simulink model "pwm_test"  (R2021b)
settings: Solver=VariableStepAuto  StartTime=0.0  StopTime=0.01  RelTol=1e-3
libraries: spsOnDelayLib x14, simulink x13
settings Model: SimulationMode=accelerator  PacingRate=1000  Creator=phddk  LastModifiedBy=phddk

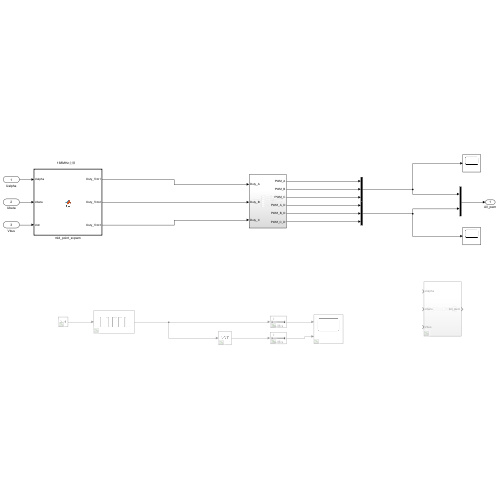
[thumbnail: Simulink's stored preview of the top-level diagram]
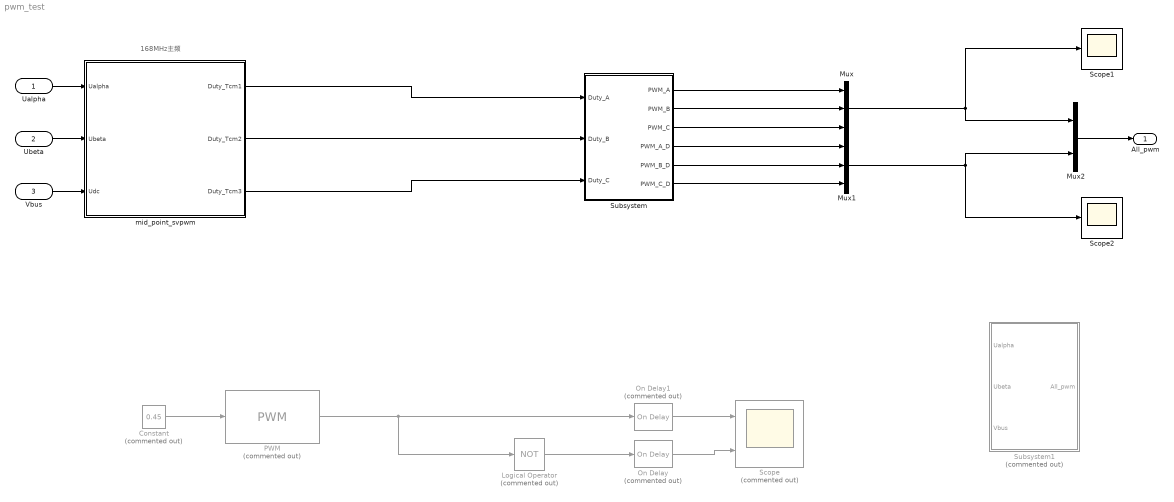
== system pwm_test ==
  note: 168MHz主频
  Ualpha : Inport
  Ubeta : Inport  Port=2
  Vbus : Inport  Port=3
  Constant : Constant  Commented=on  Value=0.45
  Logical Operator : Logic  Commented=on  Operator=NOT  AllPortsSameDT=off  OutDataTypeStr=boolean
  Mux : Mux  Inputs=3
  Mux1 : Mux  Inputs=3
  Mux2 : Mux  Inputs=2
  On Delay : spsOnDelayLib/On Delay  Commented=on  DelayType=On delay  delay=5e-6  ic=0  Ts=0
      settings: SourceProductBaseCode=PS
  On Delay1 : spsOnDelayLib/On Delay  Commented=on  DelayType=On delay  delay=5e-6  ic=0  Ts=0
      settings: SourceProductBaseCode=PS
  PWM : simulink/Discontinuities/PWM  Commented=on  DisableCoverage=on  Period=5e-4  DisallowZeroDutyCycle=off  RunAtFixedTimeIntervals=on  SampleTime=5e-5
  Scope : Scope  Commented=on  NumInputPorts=2
  Scope1 : Scope
  Scope2 : Scope
  Subsystem : Subsystem
  Subsystem1 : Subsystem  Commented=on
  mid_point_svpwm : MATLAB Function  TreatAsAtomicUnit=on
  All_pwm : Outport
  wires:
  On Delay1/1 -> Scope/1
  On Delay/1 -> Scope/2
  Logical Operator/1 -> On Delay/1
  Constant/1 -> PWM/1
  PWM/1 -> Logical Operator/1, On Delay1/1
  mid_point_svpwm/1(Duty_Tcm1) -> Subsystem/1(Duty_A)
  mid_point_svpwm/2(Duty_Tcm2) -> Subsystem/2(Duty_B)
  mid_point_svpwm/3(Duty_Tcm3) -> Subsystem/3(Duty_C)
  Mux/1 -> Mux2/1, Scope1/1
  Subsystem/1(PWM_A) -> Mux/1
  Subsystem/2(PWM_B) -> Mux/2
  Subsystem/3(PWM_C) -> Mux/3
  Subsystem/4(PWM_A_D) -> Mux1/1
  Subsystem/5(PWM_B_D) -> Mux1/2
  Subsystem/6(PWM_C_D) -> Mux1/3
  Mux1/1 -> Scope2/1, Mux2/2
  Mux2/1 -> All_pwm/1
  Ualpha/1 -> mid_point_svpwm/1(Ualpha)
  Ubeta/1 -> mid_point_svpwm/2(Ubeta)
  Vbus/1 -> mid_point_svpwm/3(Udc)

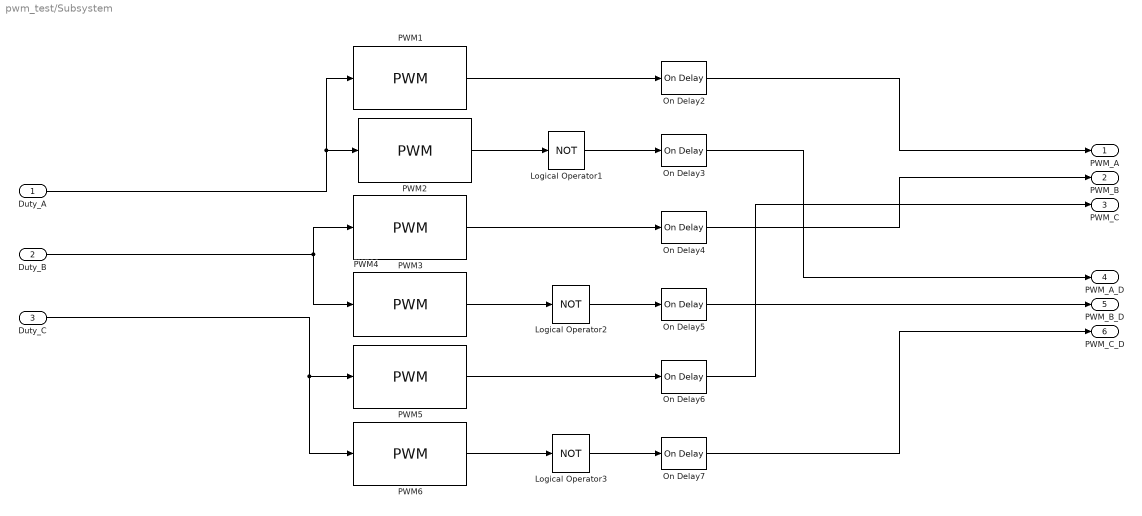
== system pwm_test/Subsystem ==
  Duty_A : Inport
  Duty_B : Inport  Port=2
  Duty_C : Inport  Port=3
  Logical Operator1 : Logic  Operator=NOT  AllPortsSameDT=off  OutDataTypeStr=boolean
  Logical Operator2 : Logic  Operator=NOT  AllPortsSameDT=off  OutDataTypeStr=boolean
  Logical Operator3 : Logic  Operator=NOT  AllPortsSameDT=off  OutDataTypeStr=boolean
  On Delay{2..7} (6 alike) : spsOnDelayLib/On Delay  DelayType=On delay  delay=5e-6  ic=0  Ts=0
      settings: SourceProductBaseCode=PS
  PWM{1..6} (6 alike) : simulink/Discontinuities/PWM  DisableCoverage=on  Period=5e-4  DisallowZeroDutyCycle=off  RunAtFixedTimeIntervals=on  SampleTime=5e-5
  PWM_A : Outport
  PWM_B : Outport  Port=2
  PWM_C : Outport  Port=3
  PWM_A_D : Outport  Port=4
  PWM_B_D : Outport  Port=5
  PWM_C_D : Outport  Port=6
  wires:
  Logical Operator1/1 -> On Delay3/1
  PWM4/1 -> Logical Operator2/1
  Logical Operator2/1 -> On Delay5/1
  Logical Operator3/1 -> On Delay7/1
  PWM6/1 -> Logical Operator3/1
  PWM2/1 -> Logical Operator1/1
  PWM3/1 -> On Delay4/1
  PWM1/1 -> On Delay2/1
  On Delay2/1 -> PWM_A/1
  Duty_A/1 -> PWM1/1, PWM2/1
  Duty_C/1 -> PWM6/1, PWM5/1
  Duty_B/1 -> PWM3/1, PWM4/1
  PWM5/1 -> On Delay6/1
  On Delay4/1 -> PWM_B/1
  On Delay6/1 -> PWM_C/1
  On Delay5/1 -> PWM_B_D/1
  On Delay7/1 -> PWM_C_D/1
  On Delay3/1 -> PWM_A_D/1

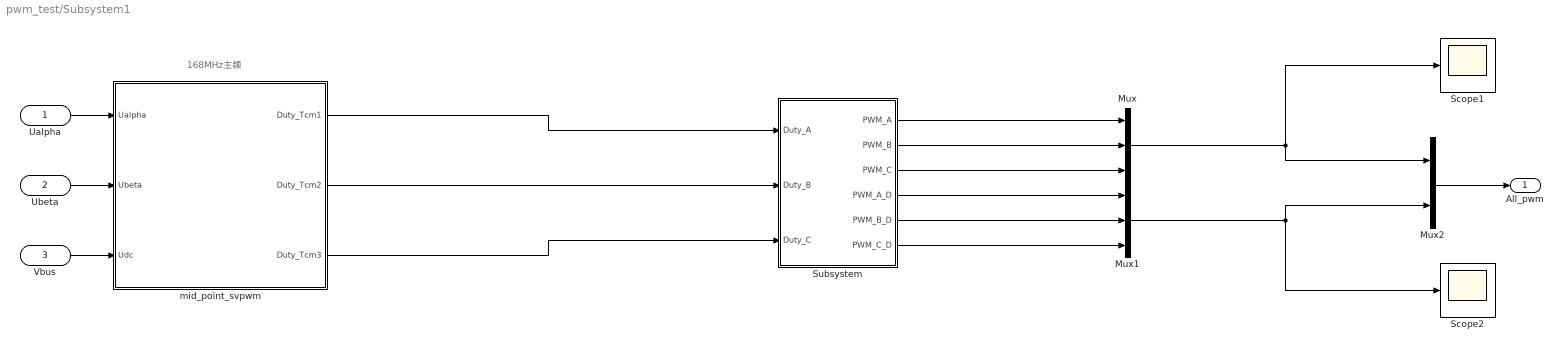
== system pwm_test/Subsystem1 ==
  note: 168MHz主频
  Ualpha : Inport
  Ubeta : Inport  Port=2
  Vbus : Inport  Port=3
  Mux : Mux  Inputs=3
  Mux1 : Mux  Inputs=3
  Mux2 : Mux  Inputs=2
  Scope1 : Scope
  Scope2 : Scope
  Subsystem : Subsystem
  mid_point_svpwm : MATLAB Function  TreatAsAtomicUnit=on
  All_pwm : Outport
  wires:
  Ubeta/1 -> mid_point_svpwm/2(Ubeta)
  Mux2/1 -> All_pwm/1
  Mux/1 -> Mux2/1, Scope1/1
  Subsystem/3(PWM_C) -> Mux/3
  Mux1/1 -> Scope2/1, Mux2/2
  mid_point_svpwm/1(Duty_Tcm1) -> Subsystem/1(Duty_A)
  mid_point_svpwm/2(Duty_Tcm2) -> Subsystem/2(Duty_B)
  mid_point_svpwm/3(Duty_Tcm3) -> Subsystem/3(Duty_C)
  Subsystem/5(PWM_B_D) -> Mux1/2
  Ualpha/1 -> mid_point_svpwm/1(Ualpha)
  Vbus/1 -> mid_point_svpwm/3(Udc)
  Subsystem/4(PWM_A_D) -> Mux1/1
  Subsystem/1(PWM_A) -> Mux/1
  Subsystem/6(PWM_C_D) -> Mux1/3
  Subsystem/2(PWM_B) -> Mux/2

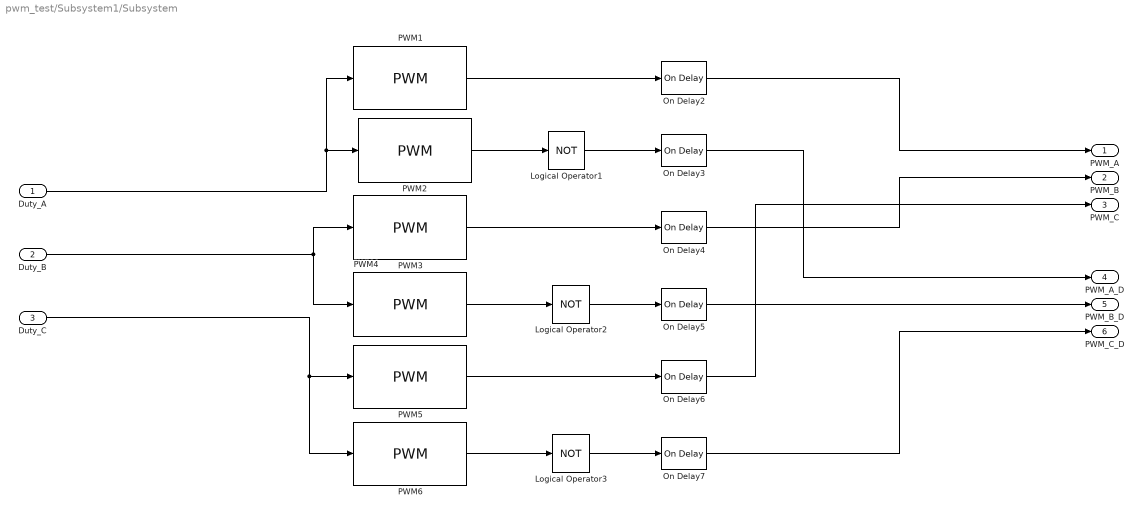
== system pwm_test/Subsystem1/Subsystem ==
  Duty_A : Inport
  Duty_B : Inport  Port=2
  Duty_C : Inport  Port=3
  Logical Operator1 : Logic  Operator=NOT  AllPortsSameDT=off  OutDataTypeStr=boolean
  Logical Operator2 : Logic  Operator=NOT  AllPortsSameDT=off  OutDataTypeStr=boolean
  Logical Operator3 : Logic  Operator=NOT  AllPortsSameDT=off  OutDataTypeStr=boolean
  On Delay{2..7} (6 alike) : spsOnDelayLib/On Delay  DelayType=On delay  delay=5e-6  ic=0  Ts=0
      settings: SourceProductBaseCode=PS
  PWM{1..6} (6 alike) : simulink/Discontinuities/PWM  DisableCoverage=on  Period=5e-4  DisallowZeroDutyCycle=off  RunAtFixedTimeIntervals=on  SampleTime=5e-5
  PWM_A : Outport
  PWM_B : Outport  Port=2
  PWM_C : Outport  Port=3
  PWM_A_D : Outport  Port=4
  PWM_B_D : Outport  Port=5
  PWM_C_D : Outport  Port=6
  wires:
  Logical Operator1/1 -> On Delay3/1
  PWM4/1 -> Logical Operator2/1
  Logical Operator2/1 -> On Delay5/1
  Logical Operator3/1 -> On Delay7/1
  PWM6/1 -> Logical Operator3/1
  PWM2/1 -> Logical Operator1/1
  PWM3/1 -> On Delay4/1
  PWM1/1 -> On Delay2/1
  On Delay2/1 -> PWM_A/1
  Duty_A/1 -> PWM1/1, PWM2/1
  Duty_C/1 -> PWM6/1, PWM5/1
  Duty_B/1 -> PWM3/1, PWM4/1
  PWM5/1 -> On Delay6/1
  On Delay4/1 -> PWM_B/1
  On Delay6/1 -> PWM_C/1
  On Delay5/1 -> PWM_B_D/1
  On Delay7/1 -> PWM_C_D/1
  On Delay3/1 -> PWM_A_D/1

== matlab function pwm_test/mid_point_svpwm ==
  data: Ualpha input; Duty_Tcm1 output; Ubeta input; Udc input; Duty_Tcm2 output; Duty_Tcm3 output
function [Duty_Tcm1,Duty_Tcm2,Duty_Tcm3] = fcn(Ualpha,Ubeta,Udc)
Tcm1 = 0;
Tcm2 = 0;
Tcm3 = 0;

Duty_Tcm1 = 0;
Duty_Tcm2 = 0;
Duty_Tcm3 = 0;


Vmax_pu=0;
Vmin_pu=0;
Vcom_pu=0;

Valpha_pu = Ualpha/Udc;
Vbeta_pu = Ubeta/Udc;
	
Va_tmp = 0.5 * Valpha_pu;
Vb_tmp = 0.8660254038 * Vbeta_pu;

Va_pu = Valpha_pu;
Vb_pu = -Va_tmp + Vb_tmp;						
Vc_pu = -Va_tmp - Vb_tmp;						

if(Va_pu > Vb_pu)
    Vmax_pu = Va_pu;
    Vmin_pu = Vb_pu;
end

if(Va_pu <= Vb_pu)
    Vmax_pu = Vb_pu;
    Vmin_pu = Va_pu;
end

if(Vc_pu > Vmax_pu)
    Vmax_pu = Vc_pu;
end
if(Vc_pu < Vmin_pu)
    Vmin_pu = Vc_pu;
end

Vcom_pu = 0.5 * (Vmax_pu + Vmin_pu);			
	
Tcm1 = (Va_pu - Vcom_pu);
Tcm2 = (Vb_pu - Vcom_pu);
Tcm3 = (Vc_pu - Vcom_pu);

if(Tcm1 > 0.5)
    Tcm1 = 0.5;
end
if(Tcm1 < -0.5)
    Tcm1 = -0.5;
end


if(Tcm2 > 0.5)
    Tcm2 = 0.5;
end
if(Tcm2 < -0.5)
    Tcm2 = -0.5;
end


if(Tcm3 > 0.5)
    Tcm3 = 0.5;
end
if(Tcm3 < -0.5)
    Tcm3 = -0.5;
end

Duty_Tcm1 = Tcm1 + 0.5;
Duty_Tcm2 = Tcm2 + 0.5;
Duty_Tcm3 = Tcm3 + 0.5;

== matlab function pwm_test/Subsystem1/mid_point_svpwm ==
  data: Ualpha input; Duty_Tcm1 output; Ubeta input; Udc input; Duty_Tcm2 output; Duty_Tcm3 output
function [Duty_Tcm1,Duty_Tcm2,Duty_Tcm3] = fcn(Ualpha,Ubeta,Udc)
Tcm1 = 0;
Tcm2 = 0;
Tcm3 = 0;

Duty_Tcm1 = 0;
Duty_Tcm2 = 0;
Duty_Tcm3 = 0;


Vmax_pu=0;
Vmin_pu=0;
Vcom_pu=0;

Valpha_pu = Ualpha/Udc;
Vbeta_pu = Ubeta/Udc;
	
Va_tmp = 0.5 * Valpha_pu;
Vb_tmp = 0.8660254038 * Vbeta_pu;

Va_pu = Valpha_pu;
Vb_pu = -Va_tmp + Vb_tmp;						
Vc_pu = -Va_tmp - Vb_tmp;						

if(Va_pu > Vb_pu)
    Vmax_pu = Va_pu;
    Vmin_pu = Vb_pu;
end

if(Va_pu <= Vb_pu)
    Vmax_pu = Vb_pu;
    Vmin_pu = Va_pu;
end

if(Vc_pu > Vmax_pu)
    Vmax_pu = Vc_pu;
end
if(Vc_pu < Vmin_pu)
    Vmin_pu = Vc_pu;
end

Vcom_pu = 0.5 * (Vmax_pu + Vmin_pu);			
	
Tcm1 = (Va_pu - Vcom_pu);
Tcm2 = (Vb_pu - Vcom_pu);
Tcm3 = (Vc_pu - Vcom_pu);

if(Tcm1 > 0.5)
    Tcm1 = 0.5;
end
if(Tcm1 < -0.5)
    Tcm1 = -0.5;
end


if(Tcm2 > 0.5)
    Tcm2 = 0.5;
end
if(Tcm2 < -0.5)
    Tcm2 = -0.5;
end


if(Tcm3 > 0.5)
    Tcm3 = 0.5;
end
if(Tcm3 < -0.5)
    Tcm3 = -0.5;
end

Duty_Tcm1 = Tcm1 + 0.5;
Duty_Tcm2 = Tcm2 + 0.5;
Duty_Tcm3 = Tcm3 + 0.5;
